simulink model "Model"  (R2023b)
settings: Solver=VariableStepAuto  StartTime=0.0  StopTime=20  RelTol=1e-3
InitFcn:
  | Parameters
values from neighbouring files (symbols this model uses):
  Area = 0.1    [Parameters.m]
  C_d = 1.05    [Parameters.m]
  cg_pos = [0.0 0 0.7]    [Parameters.m]
  ct_pos = [0 0 0.2]    [Parameters.m]
  Mass = 5    [Parameters.m]
undefined symbols (not defined in the file or in its folder): Continuous, R, Time
libraries: slpidlib x6, simulink_extras x5, sharedtransform x2, ctrlSharedLib x1, aerolibanim x1, shared6dof x1, vrlib x1, matrix_library x1
settings Model: Creator=zbyss  LastModifiedBy=zbyss

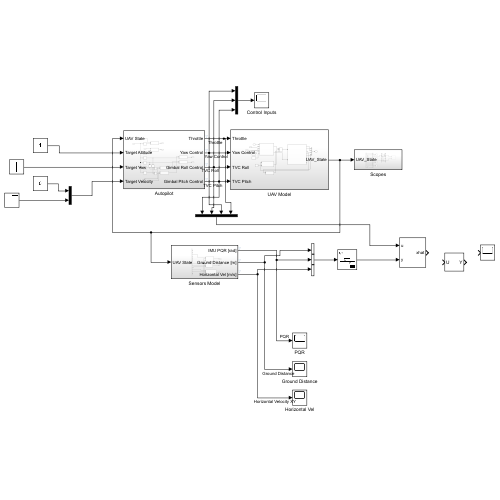
[thumbnail: Simulink's stored preview of the top-level diagram]
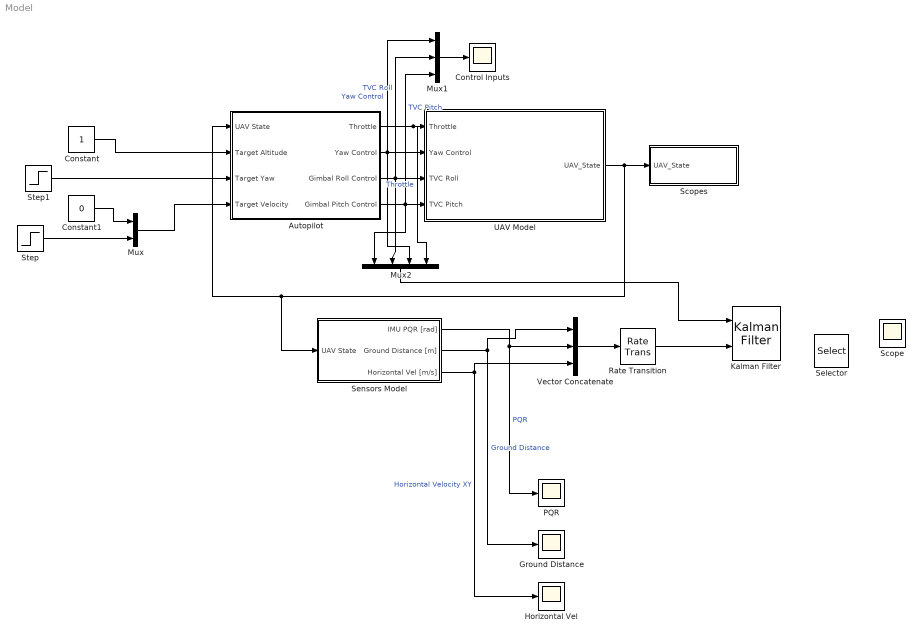
== system Model ==
  Autopilot : Subsystem
  Constant : Constant
  Constant1 : Constant  Value=0
  Control Inputs : Scope
  Ground Distance : Scope
  Horizontal Vel : Scope
  Kalman Filter : ctrlSharedLib/Kalman Filter  TimeDomain=Continuous-Time  UseCurrentEstimator=on  ModelSource=LTI State-Space Variable  ModelSourceVariable=UAV_ss  A=0.95  B=1  C=1  D=0  NumberOfStates=1  NumberOfInputs=1  NumberOfOutputs=1  InitialEstimateSource=Dialog  X0=0  P0=10  UseK=off  UseGH=off  NumberOfProcessNoiseInputs=1  G=1  TimeInvariantG=on  H=0  TimeInvariantH=on  Q=Q  TimeInvariantQ=on  R=R  TimeInvariantR=on  N=0  TimeInvariantN=on  AddInputPort=on  AddEnablePort=off  OutputEstimatedY=off  OutputP=off  Ts=-1
  Mux : Mux  Inputs=2
  Mux1 : Mux  Inputs=3
  Mux2 : Mux
  PQR : Scope
  Rate Transition : RateTransition
  Scope : Scope
  Scopes : Subsystem
  Selector : Selector  InputPortWidth=16  IndexOptions=Index vector (dialog)  Indices=[1 3]  OutputSizes=1
  Sensors Model : Subsystem
  Step : Step  Time=10  Before=-0.5  SampleTime=0
  Step1 : Step  Time=10  After=0  SampleTime=0
  UAV Model : Subsystem
  Vector Concatenate : Concatenate  NumInputs=3
  wires:
  Autopilot/1(Throttle) -> Mux2/4, UAV Model/1(Throttle)  "Throttle"
  Autopilot/2(Yaw Control) -> UAV Model/2(Yaw Control), Mux2/3, Mux1/1  "Yaw Control"
  Autopilot/3(Gimbal Roll Control) -> Mux2/2, Mux1/2, UAV Model/3(TVC Roll)  "TVC Roll"
  Autopilot/4(Gimbal Pitch Control) -> Mux2/1, Mux1/3, UAV Model/4(TVC Pitch)  "TVC Pitch"
  UAV Model/1(UAV_State) -> Sensors Model/1(UAV State), Autopilot/1(UAV State), Scopes/1(UAV_State)
  Constant/1 -> Autopilot/2(Target Altitude)
  Constant1/1 -> Mux/1
  Step/1 -> Mux/2
  Mux/1 -> Autopilot/4(Target Velocity)
  Sensors Model/1(IMU PQR [rad]) -> Vector Concatenate/2, PQR/1  "PQR"
  Sensors Model/2(Ground Distance [m]) -> Vector Concatenate/1, Ground Distance/1  "Ground Distance"
  Sensors Model/3(Horizontal Vel [m/s]) -> Vector Concatenate/3, Horizontal Vel/1  "Horizontal Velocity XY"
  Mux1/1 -> Control Inputs/1
  Step1/1 -> Autopilot/3(Target Yaw)
  Vector Concatenate/1 -> Rate Transition/1
  Mux2/1 -> Kalman Filter/1
  Rate Transition/1 -> Kalman Filter/2

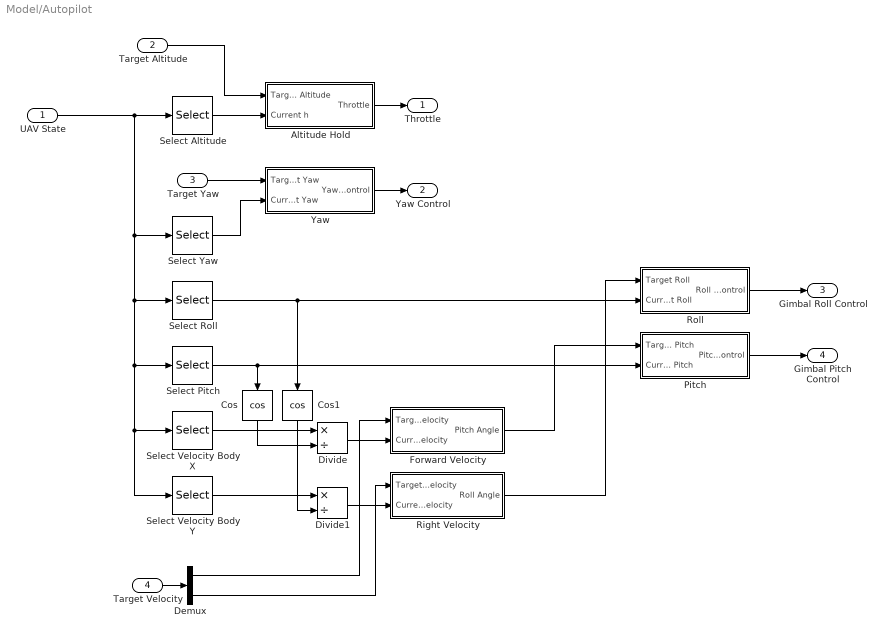
== system Model/Autopilot ==
  UAV State : Inport
  Target Altitude : Inport  Port=2
  Target Yaw : Inport  Port=3
  Target Velocity : Inport  Port=4
  Altitude Hold : Subsystem
  Cos : Trigonometry  Operator=cos
  Cos1 : Trigonometry  Operator=cos
  Demux : Demux  Outputs=2
  Divide : Product  Inputs=*/
  Divide1 : Product  Inputs=*/
  Forward Velocity : Subsystem
  Pitch : Subsystem
  Right Velocity : Subsystem
  Roll : Subsystem
  Select Altitude : Selector  InputPortWidth=12  IndexOptions=Index vector (dialog)  Indices=[3]  OutputSizes=1
  Select Pitch : Selector  InputPortWidth=12  IndexOptions=Index vector (dialog)  Indices=[8]  OutputSizes=1
  Select Roll : Selector  InputPortWidth=12  IndexOptions=Index vector (dialog)  Indices=[7]  OutputSizes=1
  Select Velocity Body X : Selector  InputPortWidth=12  IndexOptions=Index vector (dialog)  Indices=[10]  OutputSizes=1
  Select Velocity Body Y : Selector  InputPortWidth=12  IndexOptions=Index vector (dialog)  Indices=[11]  OutputSizes=1
  Select Yaw : Selector  InputPortWidth=12  IndexOptions=Index vector (dialog)  Indices=[9]  OutputSizes=1
  Yaw : Subsystem
  Throttle : Outport
  Yaw Control : Outport  Port=2
  Gimbal Roll Control : Outport  Port=3
  Gimbal Pitch Control : Outport  Port=4
  wires:
  Target Altitude/1 -> Altitude Hold/1(Target Altitude)
  Select Altitude/1 -> Altitude Hold/2(Current h)
  UAV State/1 -> Select Roll/1, Select Velocity Body Y/1, Select Velocity Body X/1, Select Pitch/1, Select Yaw/1, Select Altitude/1
  Altitude Hold/1(Throttle) -> Throttle/1
  Target Yaw/1 -> Yaw/1(Target Yaw)
  Select Yaw/1 -> Yaw/2(Current Yaw)
  Yaw/1(Yaw Control) -> Yaw Control/1
  Pitch/1(Pitch Control) -> Gimbal Pitch Control/1
  Select Pitch/1 -> Cos/1, Pitch/2(Current Pitch)
  Roll/1(Roll Control) -> Gimbal Roll Control/1
  Select Roll/1 -> Cos1/1, Roll/2(Current Roll)
  Target Velocity/1 -> Demux/1
  Select Velocity Body X/1 -> Divide/1
  Cos/1 -> Divide/2
  Divide/1 -> Forward Velocity/2(Current Velocity)
  Demux/1 -> Forward Velocity/1(Target Velocity)
  Forward Velocity/1(Pitch Angle) -> Pitch/1(Target Pitch)
  Right Velocity/1(Roll Angle) -> Roll/1(Target Roll)
  Demux/2 -> Right Velocity/1(Target Velocity)
  Divide1/1 -> Right Velocity/2(Current Velocity)
  Select Velocity Body Y/1 -> Divide1/1
  Cos1/1 -> Divide1/2

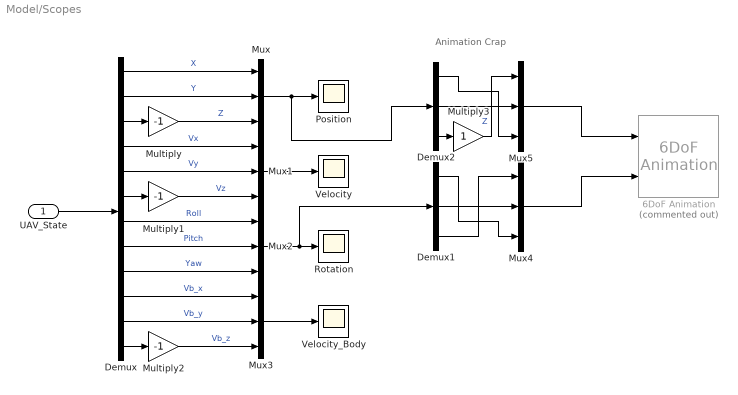
== system Model/Scopes ==
  note: Animation Crap
  UAV_State : Inport
  6DoF Animation : aerolibanim/6DoF Animation  Commented=on  u1=[-50 50 -50 50 -50 50]  u2=0.1  u3=1.0  u4=[10 0 0]  u5=Fly alongside  u6=[1 0 10]  u7=10  u8=on
  Demux : Demux  Outputs=12
  Demux1 : Demux  Outputs=3
  Demux2 : Demux  Outputs=3
  Multiply : Gain  Gain=-1
  Multiply1 : Gain  Gain=-1
  Multiply2 : Gain  Gain=-1
  Multiply3 : Gain
  Mux{,1..5} (6 alike) : Mux  Inputs=3
  Position : Scope
  Rotation : Scope
  Velocity : Scope
  Velocity_Body : Scope
  wires:
  UAV_State/1 -> Demux/1
  Demux/1 -> Mux/1  "X"
  Demux/2 -> Mux/2  "Y"
  Demux/3 -> Multiply/1
  Mux/1 -> Demux2/1, Position/1
  Demux/4 -> Mux1/1  "Vx"
  Demux/5 -> Mux1/2  "Vy"
  Demux/6 -> Multiply1/1
  Mux1/1 -> Velocity/1
  Demux/7 -> Mux2/1  "Roll"
  Demux/8 -> Mux2/2  "Pitch"
  Demux/9 -> Mux2/3  "Yaw"
  Multiply/1 -> Mux/3  "Z"
  Multiply1/1 -> Mux1/3  "Vz"
  Mux3/1 -> Velocity_Body/1
  Demux/12 -> Multiply2/1
  Multiply2/1 -> Mux3/3  "Vb_z"
  Demux/11 -> Mux3/2  "Vb_y"
  Demux/10 -> Mux3/1  "Vb_x"
  Mux2/1 -> Demux1/1, Rotation/1
  Mux4/1 -> 6DoF Animation/2
  Demux1/3 -> Mux4/1
  Demux1/2 -> Mux4/2
  Demux1/1 -> Mux4/3
  Demux2/2 -> Mux5/2
  Demux2/1 -> Mux5/3
  Demux2/3 -> Multiply3/1
  Multiply3/1 -> Mux5/1  "Z"
  Mux5/1 -> 6DoF Animation/1

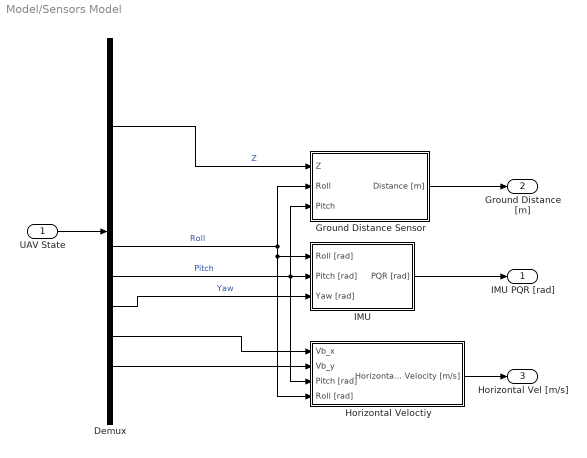
== system Model/Sensors Model ==
  UAV State : Inport
  Demux : Demux  Outputs=12
  Ground Distance Sensor : Subsystem
  Horizontal Veloctiy : Subsystem
  IMU : Subsystem
  IMU PQR [rad] : Outport
  Ground Distance [m] : Outport  Port=2
  Horizontal Vel [m/s] : Outport  Port=3
  wires:
  UAV State/1 -> Demux/1
  Demux/7 -> Horizontal Veloctiy/4(Roll [rad]), IMU/1(Roll [rad]), Ground Distance Sensor/2(Roll)  "Roll"
  Demux/8 -> Horizontal Veloctiy/3(Pitch [rad]), Ground Distance Sensor/3(Pitch), IMU/2(Pitch [rad])  "Pitch"
  Demux/9 -> IMU/3(Yaw [rad])  "Yaw"
  IMU/1(PQR [rad]) -> IMU PQR [rad]/1
  Demux/3 -> Ground Distance Sensor/1(Z)  "Z"
  Ground Distance Sensor/1(Distance [m]) -> Ground Distance [m]/1
  Demux/10 -> Horizontal Veloctiy/1(Vb_x)
  Demux/11 -> Horizontal Veloctiy/2(Vb_y)
  Horizontal Veloctiy/1(Horizontal Velocity [m/s]) -> Horizontal Vel [m/s]/1

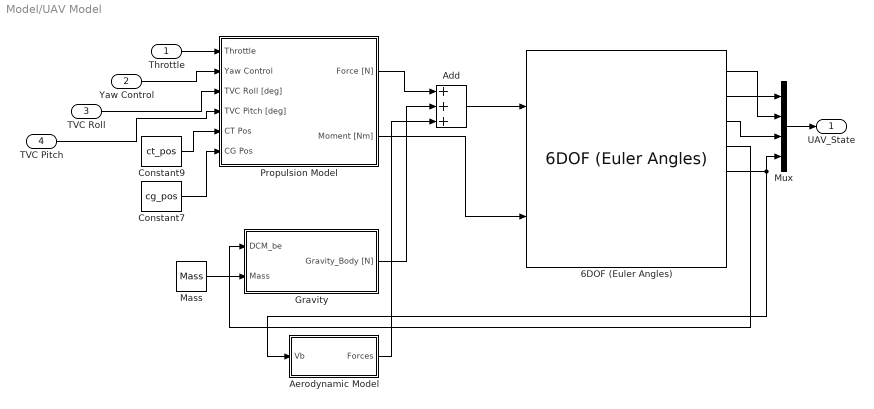
== system Model/UAV Model ==
  Throttle : Inport
  Yaw Control : Inport  Port=2
  TVC Roll : Inport  Port=3
  TVC Pitch : Inport  Port=4
  6DOF (Euler Angles) : shared6dof/6DOF (Euler Angles)  units=Metric (MKS)  mtype=Fixed  rep=Euler Angles  xme_0=[0 0 0]  Vm_0=[0 0 0]  eul_0=[0 0 0]  pm_0=[0 0 0]  mass_0=Mass  mass_e=0.5  mass_f=2.0  inertia=eye(3)  inertia_e=eye(3)  inertia_f=2*eye(3)  k_quat=1.0  vre_flag=on  abi_flag=off  aMode=0  xme_statename=''  Vm_statename=''  eul_statename=''  quat_statename=''  pm_statename=''  mass_statename=''
  Add : Sum  Inputs=+++
  Aerodynamic Model : Subsystem
  Constant7 : Constant  Value=cg_pos
  Constant9 : Constant  Value=ct_pos
  Gravity : Subsystem
  Mass : Constant  Value=Mass
  Mux : Mux
  Propulsion Model : Subsystem
  UAV_State : Outport
  wires:
  Propulsion Model/1(Force [N]) -> Add/1
  Add/1 -> 6DOF (Euler Angles)/1
  TVC Roll/1 -> Propulsion Model/3(TVC Roll [deg])
  Throttle/1 -> Propulsion Model/1(Throttle)
  Gravity/1(Gravity_Body [N]) -> Add/2
  Propulsion Model/2(Moment [Nm]) -> 6DOF (Euler Angles)/2
  Constant9/1 -> Propulsion Model/5(CT Pos)
  Constant7/1 -> Propulsion Model/6(CG Pos)
  Mass/1 -> Gravity/2(Mass)
  6DOF (Euler Angles)/4 -> Gravity/1(DCM_be)
  Yaw Control/1 -> Propulsion Model/2(Yaw Control)
  6DOF (Euler Angles)/3 -> Mux/3
  6DOF (Euler Angles)/2 -> Mux/1
  Mux/1 -> UAV_State/1
  TVC Pitch/1 -> Propulsion Model/4(TVC Pitch [deg])
  6DOF (Euler Angles)/1 -> Mux/2
  6DOF (Euler Angles)/5 -> Aerodynamic Model/1(Vb), Mux/4
  Aerodynamic Model/1(Forces) -> Add/3

== system Model/Autopilot/Altitude Hold ==
  Target Altitude : Inport
  Current h : Inport  Port=2
  Altitude Hold PID : slpidlib/PID Controller  Controller=PID  Form=Parallel  TimeDomain=Continuous-time  UseExternalTs=off  SampleTime=-1  IntegratorMethod=Forward Euler  FilterMethod=Forward Euler  ControllerParametersSource=internal  P=1.20920987907462  I=0.107771167125322  UseKiTs=off  D=3.01454491123333  N=1745.9050909753  UseFilter=on  TunerSelectOption=Transfer Function Based (PID Tuner App)  InitialConditionSource=internal  InitialConditionForIntegrator=0  InitialConditionForFilter=0  DifferentiatorICPrevScaledInput=0  ExternalReset=none  TrackingMode=off  Kt=1  LimitOutput=off  SatLimitsSource=internal  UpperSaturationLimit=inf  LowerSaturationLimit=-inf  LinearizeAsGain=on  AntiWindupMode=none  Kb=1  LimitIntegrator=off  UpperIntegratorSaturationLimit=inf  LowerIntegratorSaturationLimit=-inf  POutMin=[]  POutMax=[]  IOutMin=[]  IOutMax=[]  DOutMin=[]  DOutMax=[]  NOutMin=[]  NOutMax=[]  SumOutMin=[]  SumOutMax=[]  SaturationOutMin=[]  SaturationOutMax=[]  PParamMin=[]  PParamMax=[]  IParamMin=[]  IParamMax=[]  DParamMin=[]  DParamMax=[]  NParamMin=[]  NParamMax=[]  KbParamMin=[]  KbParamMax=[]  KtParamMin=[]  KtParamMax=[]  KbOutMin=[]  KbOutMax=[]  KtOutMin=[]  KtOutMax=[]  IntegratorOutMin=[]  IntegratorOutMax=[]  FilterOutMin=[]  FilterOutMax=[]  SumI1OutMin=[]  SumI1OutMax=[]  SumI2OutMin=[]  SumI2OutMax=[]  SumI3OutMin=[]  SumI3OutMax=[]  SumI4OutMin=[]  SumI4OutMax=[]  SumDOutMin=[]  SumDOutMax=[]  DifferentiatorOutMin=[]  DifferentiatorOutMax=[]  FilterDiffOutCoefMin=[]  FilterDiffOutCoefMax=[]  ReciprocalOutMin=[]  ReciprocalOutMax=[]  SumDenOutMin=[]  SumDenOutMax=[]  SumNumOutMin=[]  SumNumOutMax=[]  DivideOutMin=[]  DivideOutMax=[]  UdiffTsProdOutMin=[]  UdiffTsProdOutMax=[]  NTsProdOutMin=[]  NTsProdOutMax=[]  UintegralTsProdOutMin=[]  UintegralTsProdOutMax=[]  UngainTsProdOutMin=[]  UngainTsProdOutMax=[]  ClampingZeroOutDataTypeStr=Inherit: Inherit via back propagation  ClampingZeroOutMin=[]  ClampingZeroOutMax=[]  FilterDenConstantOutDataTypeStr=Inherit: Inherit via back propagation  FilterDenConstantOutMin=[]  FilterDenConstantOutMax=[]  PCopyOutDataTypeStr=Inherit: Inherit via back propagation  PCopyOutMin=[]  PCopyOutMax=[]  NCopyOutDataTypeStr=Inherit: Inherit via back propagation  NCopyOutMin=[]  NCopyOutMax=[]  IntegratorContinuousStateAttributes=''  IntegratorStateMustResolveToSignalObject=off  IntegratorRTWStateStorageClass=Auto  FilterContinuousStateAttributes=''  FilterStateMustResolveToSignalObject=off  FilterRTWStateStorageClass=Auto  ParallelPVariant=InternalParameters  IdealPVariant=Disabled  IVariant=InternalParameters  DVariant=InternalParameters  IntegratorVariant=Continuous  SatVariant=Disabled  AWVariant=Passthrough  PCopyVariant=Disabled  TRVariant=Disabled  FdbkBlocksVariant=Forward  IdealPFdbkVariant=Disabled  SatFdbkVariant=Disabled  DerivativeFilterVariant=ContFilter  NVariant=InternalParameters  NCopyVariant=Disabled  FilterICVariant=InternalICsFilter  IntegratorICVariant=InternalICs  ExternalResetVariant=Disabled  TRSumVariant=Passthrough  SumFdbkVariant=Disabled  SumVariant=Sum_PID  TsampFilterVariant=InternalTs  TsampNgainVariant=Passthrough  TsampIntegralVariant=Disabled_SignalSpec  ExternalSaturationOutDataTypeStr=Inherit: Same as second input
  Multiply : Gain  Gain=-1
  Saturation : Saturate  UpperLimit=1  LowerLimit=0
  Sum : Sum  Inputs=|+-
  Throttle : Outport
  wires:
  Sum/1 -> Altitude Hold PID/1
  Target Altitude/1 -> Sum/1
  Current h/1 -> Multiply/1
  Altitude Hold PID/1 -> Saturation/1
  Multiply/1 -> Sum/2
  Saturation/1 -> Throttle/1

== system Model/Autopilot/Forward Velocity ==
  Target Velocity : Inport
  Current Velocity : Inport  Port=2
  Gain : Gain  Gain=-1
  PID Controller : slpidlib/PID Controller  Controller=PID  Form=Parallel  TimeDomain=Continuous-time  UseExternalTs=off  SampleTime=-1  IntegratorMethod=Forward Euler  FilterMethod=Forward Euler  ControllerParametersSource=internal  P=5  I=1  UseKiTs=off  D=0  N=100  UseFilter=on  TunerSelectOption=Transfer Function Based (PID Tuner App)  InitialConditionSource=internal  InitialConditionForIntegrator=0  InitialConditionForFilter=0  DifferentiatorICPrevScaledInput=0  ExternalReset=none  TrackingMode=off  Kt=1  LimitOutput=off  SatLimitsSource=internal  UpperSaturationLimit=inf  LowerSaturationLimit=-inf  LinearizeAsGain=on  AntiWindupMode=none  Kb=1  LimitIntegrator=off  UpperIntegratorSaturationLimit=inf  LowerIntegratorSaturationLimit=-inf  POutMin=[]  POutMax=[]  IOutMin=[]  IOutMax=[]  DOutMin=[]  DOutMax=[]  NOutMin=[]  NOutMax=[]  SumOutMin=[]  SumOutMax=[]  SaturationOutMin=[]  SaturationOutMax=[]  PParamMin=[]  PParamMax=[]  IParamMin=[]  IParamMax=[]  DParamMin=[]  DParamMax=[]  NParamMin=[]  NParamMax=[]  KbParamMin=[]  KbParamMax=[]  KtParamMin=[]  KtParamMax=[]  KbOutMin=[]  KbOutMax=[]  KtOutMin=[]  KtOutMax=[]  IntegratorOutMin=[]  IntegratorOutMax=[]  FilterOutMin=[]  FilterOutMax=[]  SumI1OutMin=[]  SumI1OutMax=[]  SumI2OutMin=[]  SumI2OutMax=[]  SumI3OutMin=[]  SumI3OutMax=[]  SumI4OutMin=[]  SumI4OutMax=[]  SumDOutMin=[]  SumDOutMax=[]  DifferentiatorOutMin=[]  DifferentiatorOutMax=[]  FilterDiffOutCoefMin=[]  FilterDiffOutCoefMax=[]  ReciprocalOutMin=[]  ReciprocalOutMax=[]  SumDenOutMin=[]  SumDenOutMax=[]  SumNumOutMin=[]  SumNumOutMax=[]  DivideOutMin=[]  DivideOutMax=[]  UdiffTsProdOutMin=[]  UdiffTsProdOutMax=[]  NTsProdOutMin=[]  NTsProdOutMax=[]  UintegralTsProdOutMin=[]  UintegralTsProdOutMax=[]  UngainTsProdOutMin=[]  UngainTsProdOutMax=[]  ClampingZeroOutDataTypeStr=Inherit: Inherit via back propagation  ClampingZeroOutMin=[]  ClampingZeroOutMax=[]  FilterDenConstantOutDataTypeStr=Inherit: Inherit via back propagation  FilterDenConstantOutMin=[]  FilterDenConstantOutMax=[]  PCopyOutDataTypeStr=Inherit: Inherit via back propagation  PCopyOutMin=[]  PCopyOutMax=[]  NCopyOutDataTypeStr=Inherit: Inherit via back propagation  NCopyOutMin=[]  NCopyOutMax=[]  IntegratorContinuousStateAttributes=''  IntegratorStateMustResolveToSignalObject=off  IntegratorRTWStateStorageClass=Auto  FilterContinuousStateAttributes=''  FilterStateMustResolveToSignalObject=off  FilterRTWStateStorageClass=Auto  ParallelPVariant=InternalParameters  IdealPVariant=Disabled  IVariant=InternalParameters  DVariant=InternalParameters  IntegratorVariant=Continuous  SatVariant=Disabled  AWVariant=Passthrough  PCopyVariant=Disabled  TRVariant=Disabled  FdbkBlocksVariant=Forward  IdealPFdbkVariant=Disabled  SatFdbkVariant=Disabled  DerivativeFilterVariant=ContFilter  NVariant=InternalParameters  NCopyVariant=Disabled  FilterICVariant=InternalICsFilter  IntegratorICVariant=InternalICs  ExternalResetVariant=Disabled  TRSumVariant=Passthrough  SumFdbkVariant=Disabled  SumVariant=Sum_PID  TsampFilterVariant=InternalTs  TsampNgainVariant=Passthrough  TsampIntegralVariant=Disabled_SignalSpec  ExternalSaturationOutDataTypeStr=Inherit: Same as second input
  Saturation : Saturate  UpperLimit=5  LowerLimit=-5
  Sum : Sum  Inputs=|+-
  Pitch Angle : Outport
  wires:
  Target Velocity/1 -> Sum/1
  Current Velocity/1 -> Sum/2
  Sum/1 -> PID Controller/1
  PID Controller/1 -> Gain/1
  Saturation/1 -> Pitch Angle/1
  Gain/1 -> Saturation/1

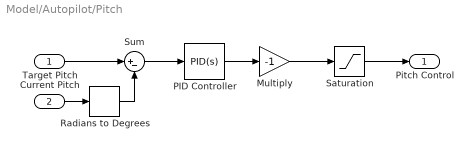
== system Model/Autopilot/Pitch ==
  Target Pitch : Inport
  Current Pitch : Inport  Port=2
  Multiply : Gain  Gain=-1
  PID Controller : slpidlib/PID Controller  Controller=PID  Form=Parallel  TimeDomain=Continuous-time  UseExternalTs=off  SampleTime=-1  IntegratorMethod=Forward Euler  FilterMethod=Forward Euler  ControllerParametersSource=internal  P=2  I=1  UseKiTs=off  D=1  N=100  UseFilter=on  TunerSelectOption=Transfer Function Based (PID Tuner App)  InitialConditionSource=internal  InitialConditionForIntegrator=0  InitialConditionForFilter=0  DifferentiatorICPrevScaledInput=0  ExternalReset=none  TrackingMode=off  Kt=1  LimitOutput=off  SatLimitsSource=internal  UpperSaturationLimit=inf  LowerSaturationLimit=-inf  LinearizeAsGain=on  AntiWindupMode=none  Kb=1  LimitIntegrator=off  UpperIntegratorSaturationLimit=inf  LowerIntegratorSaturationLimit=-inf  POutMin=[]  POutMax=[]  IOutMin=[]  IOutMax=[]  DOutMin=[]  DOutMax=[]  NOutMin=[]  NOutMax=[]  SumOutMin=[]  SumOutMax=[]  SaturationOutMin=[]  SaturationOutMax=[]  PParamMin=[]  PParamMax=[]  IParamMin=[]  IParamMax=[]  DParamMin=[]  DParamMax=[]  NParamMin=[]  NParamMax=[]  KbParamMin=[]  KbParamMax=[]  KtParamMin=[]  KtParamMax=[]  KbOutMin=[]  KbOutMax=[]  KtOutMin=[]  KtOutMax=[]  IntegratorOutMin=[]  IntegratorOutMax=[]  FilterOutMin=[]  FilterOutMax=[]  SumI1OutMin=[]  SumI1OutMax=[]  SumI2OutMin=[]  SumI2OutMax=[]  SumI3OutMin=[]  SumI3OutMax=[]  SumI4OutMin=[]  SumI4OutMax=[]  SumDOutMin=[]  SumDOutMax=[]  DifferentiatorOutMin=[]  DifferentiatorOutMax=[]  FilterDiffOutCoefMin=[]  FilterDiffOutCoefMax=[]  ReciprocalOutMin=[]  ReciprocalOutMax=[]  SumDenOutMin=[]  SumDenOutMax=[]  SumNumOutMin=[]  SumNumOutMax=[]  DivideOutMin=[]  DivideOutMax=[]  UdiffTsProdOutMin=[]  UdiffTsProdOutMax=[]  NTsProdOutMin=[]  NTsProdOutMax=[]  UintegralTsProdOutMin=[]  UintegralTsProdOutMax=[]  UngainTsProdOutMin=[]  UngainTsProdOutMax=[]  ClampingZeroOutDataTypeStr=Inherit: Inherit via back propagation  ClampingZeroOutMin=[]  ClampingZeroOutMax=[]  FilterDenConstantOutDataTypeStr=Inherit: Inherit via back propagation  FilterDenConstantOutMin=[]  FilterDenConstantOutMax=[]  PCopyOutDataTypeStr=Inherit: Inherit via back propagation  PCopyOutMin=[]  PCopyOutMax=[]  NCopyOutDataTypeStr=Inherit: Inherit via back propagation  NCopyOutMin=[]  NCopyOutMax=[]  IntegratorContinuousStateAttributes=''  IntegratorStateMustResolveToSignalObject=off  IntegratorRTWStateStorageClass=Auto  FilterContinuousStateAttributes=''  FilterStateMustResolveToSignalObject=off  FilterRTWStateStorageClass=Auto  ParallelPVariant=InternalParameters  IdealPVariant=Disabled  IVariant=InternalParameters  DVariant=InternalParameters  IntegratorVariant=Continuous  SatVariant=Disabled  AWVariant=Passthrough  PCopyVariant=Disabled  TRVariant=Disabled  FdbkBlocksVariant=Forward  IdealPFdbkVariant=Disabled  SatFdbkVariant=Disabled  DerivativeFilterVariant=ContFilter  NVariant=InternalParameters  NCopyVariant=Disabled  FilterICVariant=InternalICsFilter  IntegratorICVariant=InternalICs  ExternalResetVariant=Disabled  TRSumVariant=Passthrough  SumFdbkVariant=Disabled  SumVariant=Sum_PID  TsampFilterVariant=InternalTs  TsampNgainVariant=Passthrough  TsampIntegralVariant=Disabled_SignalSpec  ExternalSaturationOutDataTypeStr=Inherit: Same as second input
  Radians to Degrees : simulink_extras/Transformations/Radians to Degrees
  Saturation : Saturate  UpperLimit=15  LowerLimit=-15
  Sum : Sum  Inputs=|+-
  Pitch Control : Outport
  wires:
  Target Pitch/1 -> Sum/1
  PID Controller/1 -> Multiply/1
  Current Pitch/1 -> Radians to Degrees/1
  Sum/1 -> PID Controller/1
  Saturation/1 -> Pitch Control/1
  Multiply/1 -> Saturation/1
  Radians to Degrees/1 -> Sum/2

== system Model/Autopilot/Right Velocity ==
  Target Velocity : Inport
  Current Velocity : Inport  Port=2
  PID Controller : slpidlib/PID Controller  Controller=PID  Form=Parallel  TimeDomain=Continuous-time  UseExternalTs=off  SampleTime=-1  IntegratorMethod=Forward Euler  FilterMethod=Forward Euler  ControllerParametersSource=internal  P=5  I=1  UseKiTs=off  D=0  N=100  UseFilter=on  TunerSelectOption=Transfer Function Based (PID Tuner App)  InitialConditionSource=internal  InitialConditionForIntegrator=0  InitialConditionForFilter=0  DifferentiatorICPrevScaledInput=0  ExternalReset=none  TrackingMode=off  Kt=1  LimitOutput=off  SatLimitsSource=internal  UpperSaturationLimit=inf  LowerSaturationLimit=-inf  LinearizeAsGain=on  AntiWindupMode=none  Kb=1  LimitIntegrator=off  UpperIntegratorSaturationLimit=inf  LowerIntegratorSaturationLimit=-inf  POutMin=[]  POutMax=[]  IOutMin=[]  IOutMax=[]  DOutMin=[]  DOutMax=[]  NOutMin=[]  NOutMax=[]  SumOutMin=[]  SumOutMax=[]  SaturationOutMin=[]  SaturationOutMax=[]  PParamMin=[]  PParamMax=[]  IParamMin=[]  IParamMax=[]  DParamMin=[]  DParamMax=[]  NParamMin=[]  NParamMax=[]  KbParamMin=[]  KbParamMax=[]  KtParamMin=[]  KtParamMax=[]  KbOutMin=[]  KbOutMax=[]  KtOutMin=[]  KtOutMax=[]  IntegratorOutMin=[]  IntegratorOutMax=[]  FilterOutMin=[]  FilterOutMax=[]  SumI1OutMin=[]  SumI1OutMax=[]  SumI2OutMin=[]  SumI2OutMax=[]  SumI3OutMin=[]  SumI3OutMax=[]  SumI4OutMin=[]  SumI4OutMax=[]  SumDOutMin=[]  SumDOutMax=[]  DifferentiatorOutMin=[]  DifferentiatorOutMax=[]  FilterDiffOutCoefMin=[]  FilterDiffOutCoefMax=[]  ReciprocalOutMin=[]  ReciprocalOutMax=[]  SumDenOutMin=[]  SumDenOutMax=[]  SumNumOutMin=[]  SumNumOutMax=[]  DivideOutMin=[]  DivideOutMax=[]  UdiffTsProdOutMin=[]  UdiffTsProdOutMax=[]  NTsProdOutMin=[]  NTsProdOutMax=[]  UintegralTsProdOutMin=[]  UintegralTsProdOutMax=[]  UngainTsProdOutMin=[]  UngainTsProdOutMax=[]  ClampingZeroOutDataTypeStr=Inherit: Inherit via back propagation  ClampingZeroOutMin=[]  ClampingZeroOutMax=[]  FilterDenConstantOutDataTypeStr=Inherit: Inherit via back propagation  FilterDenConstantOutMin=[]  FilterDenConstantOutMax=[]  PCopyOutDataTypeStr=Inherit: Inherit via back propagation  PCopyOutMin=[]  PCopyOutMax=[]  NCopyOutDataTypeStr=Inherit: Inherit via back propagation  NCopyOutMin=[]  NCopyOutMax=[]  IntegratorContinuousStateAttributes=''  IntegratorStateMustResolveToSignalObject=off  IntegratorRTWStateStorageClass=Auto  FilterContinuousStateAttributes=''  FilterStateMustResolveToSignalObject=off  FilterRTWStateStorageClass=Auto  ParallelPVariant=InternalParameters  IdealPVariant=Disabled  IVariant=InternalParameters  DVariant=InternalParameters  IntegratorVariant=Continuous  SatVariant=Disabled  AWVariant=Passthrough  PCopyVariant=Disabled  TRVariant=Disabled  FdbkBlocksVariant=Forward  IdealPFdbkVariant=Disabled  SatFdbkVariant=Disabled  DerivativeFilterVariant=ContFilter  NVariant=InternalParameters  NCopyVariant=Disabled  FilterICVariant=InternalICsFilter  IntegratorICVariant=InternalICs  ExternalResetVariant=Disabled  TRSumVariant=Passthrough  SumFdbkVariant=Disabled  SumVariant=Sum_PID  TsampFilterVariant=InternalTs  TsampNgainVariant=Passthrough  TsampIntegralVariant=Disabled_SignalSpec  ExternalSaturationOutDataTypeStr=Inherit: Same as second input
  Saturation : Saturate  UpperLimit=5  LowerLimit=-5
  Sum : Sum  Inputs=|+-
  Roll Angle : Outport
  wires:
  Target Velocity/1 -> Sum/1
  Current Velocity/1 -> Sum/2
  Sum/1 -> PID Controller/1
  PID Controller/1 -> Saturation/1
  Saturation/1 -> Roll Angle/1

== system Model/Autopilot/Roll ==
  Target Roll : Inport
  Current Roll : Inport  Port=2
  Multiply : Gain  Gain=-1
  PID Controller : slpidlib/PID Controller  Controller=PID  Form=Parallel  TimeDomain=Continuous-time  UseExternalTs=off  SampleTime=-1  IntegratorMethod=Forward Euler  FilterMethod=Forward Euler  ControllerParametersSource=internal  P=1  I=1  UseKiTs=off  D=1  N=100  UseFilter=on  TunerSelectOption=Transfer Function Based (PID Tuner App)  InitialConditionSource=internal  InitialConditionForIntegrator=0  InitialConditionForFilter=0  DifferentiatorICPrevScaledInput=0  ExternalReset=none  TrackingMode=off  Kt=1  LimitOutput=off  SatLimitsSource=internal  UpperSaturationLimit=inf  LowerSaturationLimit=-inf  LinearizeAsGain=on  AntiWindupMode=none  Kb=1  LimitIntegrator=off  UpperIntegratorSaturationLimit=inf  LowerIntegratorSaturationLimit=-inf  POutMin=[]  POutMax=[]  IOutMin=[]  IOutMax=[]  DOutMin=[]  DOutMax=[]  NOutMin=[]  NOutMax=[]  SumOutMin=[]  SumOutMax=[]  SaturationOutMin=[]  SaturationOutMax=[]  PParamMin=[]  PParamMax=[]  IParamMin=[]  IParamMax=[]  DParamMin=[]  DParamMax=[]  NParamMin=[]  NParamMax=[]  KbParamMin=[]  KbParamMax=[]  KtParamMin=[]  KtParamMax=[]  KbOutMin=[]  KbOutMax=[]  KtOutMin=[]  KtOutMax=[]  IntegratorOutMin=[]  IntegratorOutMax=[]  FilterOutMin=[]  FilterOutMax=[]  SumI1OutMin=[]  SumI1OutMax=[]  SumI2OutMin=[]  SumI2OutMax=[]  SumI3OutMin=[]  SumI3OutMax=[]  SumI4OutMin=[]  SumI4OutMax=[]  SumDOutMin=[]  SumDOutMax=[]  DifferentiatorOutMin=[]  DifferentiatorOutMax=[]  FilterDiffOutCoefMin=[]  FilterDiffOutCoefMax=[]  ReciprocalOutMin=[]  ReciprocalOutMax=[]  SumDenOutMin=[]  SumDenOutMax=[]  SumNumOutMin=[]  SumNumOutMax=[]  DivideOutMin=[]  DivideOutMax=[]  UdiffTsProdOutMin=[]  UdiffTsProdOutMax=[]  NTsProdOutMin=[]  NTsProdOutMax=[]  UintegralTsProdOutMin=[]  UintegralTsProdOutMax=[]  UngainTsProdOutMin=[]  UngainTsProdOutMax=[]  ClampingZeroOutDataTypeStr=Inherit: Inherit via back propagation  ClampingZeroOutMin=[]  ClampingZeroOutMax=[]  FilterDenConstantOutDataTypeStr=Inherit: Inherit via back propagation  FilterDenConstantOutMin=[]  FilterDenConstantOutMax=[]  PCopyOutDataTypeStr=Inherit: Inherit via back propagation  PCopyOutMin=[]  PCopyOutMax=[]  NCopyOutDataTypeStr=Inherit: Inherit via back propagation  NCopyOutMin=[]  NCopyOutMax=[]  IntegratorContinuousStateAttributes=''  IntegratorStateMustResolveToSignalObject=off  IntegratorRTWStateStorageClass=Auto  FilterContinuousStateAttributes=''  FilterStateMustResolveToSignalObject=off  FilterRTWStateStorageClass=Auto  ParallelPVariant=InternalParameters  IdealPVariant=Disabled  IVariant=InternalParameters  DVariant=InternalParameters  IntegratorVariant=Continuous  SatVariant=Disabled  AWVariant=Passthrough  PCopyVariant=Disabled  TRVariant=Disabled  FdbkBlocksVariant=Forward  IdealPFdbkVariant=Disabled  SatFdbkVariant=Disabled  DerivativeFilterVariant=ContFilter  NVariant=InternalParameters  NCopyVariant=Disabled  FilterICVariant=InternalICsFilter  IntegratorICVariant=InternalICs  ExternalResetVariant=Disabled  TRSumVariant=Passthrough  SumFdbkVariant=Disabled  SumVariant=Sum_PID  TsampFilterVariant=InternalTs  TsampNgainVariant=Passthrough  TsampIntegralVariant=Disabled_SignalSpec  ExternalSaturationOutDataTypeStr=Inherit: Same as second input
  Radians to Degrees : simulink_extras/Transformations/Radians to Degrees
  Saturation : Saturate  UpperLimit=15  LowerLimit=-15
  Sum : Sum  Inputs=|+-
  Roll Control : Outport
  wires:
  Target Roll/1 -> Sum/1
  PID Controller/1 -> Multiply/1
  Current Roll/1 -> Radians to Degrees/1
  Radians to Degrees/1 -> Sum/2
  Sum/1 -> PID Controller/1
  Saturation/1 -> Roll Control/1
  Multiply/1 -> Saturation/1

== system Model/Autopilot/Yaw ==
  Target Yaw : Inport
  Current Yaw : Inport  Port=2
  PID Controller : slpidlib/PID Controller  Controller=PID  Form=Parallel  TimeDomain=Continuous-time  UseExternalTs=off  SampleTime=-1  IntegratorMethod=Forward Euler  FilterMethod=Forward Euler  ControllerParametersSource=internal  P=0.042797411577694  I=0.000605883707407974  UseKiTs=off  D=0.5015154023923  N=234.053751783226  UseFilter=on  TunerSelectOption=Transfer Function Based (PID Tuner App)  InitialConditionSource=internal  InitialConditionForIntegrator=0  InitialConditionForFilter=0  DifferentiatorICPrevScaledInput=0  ExternalReset=none  TrackingMode=off  Kt=1  LimitOutput=off  SatLimitsSource=internal  UpperSaturationLimit=inf  LowerSaturationLimit=-inf  LinearizeAsGain=on  AntiWindupMode=none  Kb=1  LimitIntegrator=off  UpperIntegratorSaturationLimit=inf  LowerIntegratorSaturationLimit=-inf  POutMin=[]  POutMax=[]  IOutMin=[]  IOutMax=[]  DOutMin=[]  DOutMax=[]  NOutMin=[]  NOutMax=[]  SumOutMin=[]  SumOutMax=[]  SaturationOutMin=[]  SaturationOutMax=[]  PParamMin=[]  PParamMax=[]  IParamMin=[]  IParamMax=[]  DParamMin=[]  DParamMax=[]  NParamMin=[]  NParamMax=[]  KbParamMin=[]  KbParamMax=[]  KtParamMin=[]  KtParamMax=[]  KbOutMin=[]  KbOutMax=[]  KtOutMin=[]  KtOutMax=[]  IntegratorOutMin=[]  IntegratorOutMax=[]  FilterOutMin=[]  FilterOutMax=[]  SumI1OutMin=[]  SumI1OutMax=[]  SumI2OutMin=[]  SumI2OutMax=[]  SumI3OutMin=[]  SumI3OutMax=[]  SumI4OutMin=[]  SumI4OutMax=[]  SumDOutMin=[]  SumDOutMax=[]  DifferentiatorOutMin=[]  DifferentiatorOutMax=[]  FilterDiffOutCoefMin=[]  FilterDiffOutCoefMax=[]  ReciprocalOutMin=[]  ReciprocalOutMax=[]  SumDenOutMin=[]  SumDenOutMax=[]  SumNumOutMin=[]  SumNumOutMax=[]  DivideOutMin=[]  DivideOutMax=[]  UdiffTsProdOutMin=[]  UdiffTsProdOutMax=[]  NTsProdOutMin=[]  NTsProdOutMax=[]  UintegralTsProdOutMin=[]  UintegralTsProdOutMax=[]  UngainTsProdOutMin=[]  UngainTsProdOutMax=[]  ClampingZeroOutDataTypeStr=Inherit: Inherit via back propagation  ClampingZeroOutMin=[]  ClampingZeroOutMax=[]  FilterDenConstantOutDataTypeStr=Inherit: Inherit via back propagation  FilterDenConstantOutMin=[]  FilterDenConstantOutMax=[]  PCopyOutDataTypeStr=Inherit: Inherit via back propagation  PCopyOutMin=[]  PCopyOutMax=[]  NCopyOutDataTypeStr=Inherit: Inherit via back propagation  NCopyOutMin=[]  NCopyOutMax=[]  IntegratorContinuousStateAttributes=''  IntegratorStateMustResolveToSignalObject=off  IntegratorRTWStateStorageClass=Auto  FilterContinuousStateAttributes=''  FilterStateMustResolveToSignalObject=off  FilterRTWStateStorageClass=Auto  ParallelPVariant=InternalParameters  IdealPVariant=Disabled  IVariant=InternalParameters  DVariant=InternalParameters  IntegratorVariant=Continuous  SatVariant=Disabled  AWVariant=Passthrough  PCopyVariant=Disabled  TRVariant=Disabled  FdbkBlocksVariant=Forward  IdealPFdbkVariant=Disabled  SatFdbkVariant=Disabled  DerivativeFilterVariant=ContFilter  NVariant=InternalParameters  NCopyVariant=Disabled  FilterICVariant=InternalICsFilter  IntegratorICVariant=InternalICs  ExternalResetVariant=Disabled  TRSumVariant=Passthrough  SumFdbkVariant=Disabled  SumVariant=Sum_PID  TsampFilterVariant=InternalTs  TsampNgainVariant=Passthrough  TsampIntegralVariant=Disabled_SignalSpec  ExternalSaturationOutDataTypeStr=Inherit: Same as second input
  Radians to Degrees : simulink_extras/Transformations/Radians to Degrees
  Saturation : Saturate  UpperLimit=1  LowerLimit=-1
  Sum : Sum  Inputs=|+-
  Yaw Control : Outport
  wires:
  Target Yaw/1 -> Sum/1
  Sum/1 -> PID Controller/1
  PID Controller/1 -> Saturation/1
  Saturation/1 -> Yaw Control/1
  Current Yaw/1 -> Radians to Degrees/1
  Radians to Degrees/1 -> Sum/2

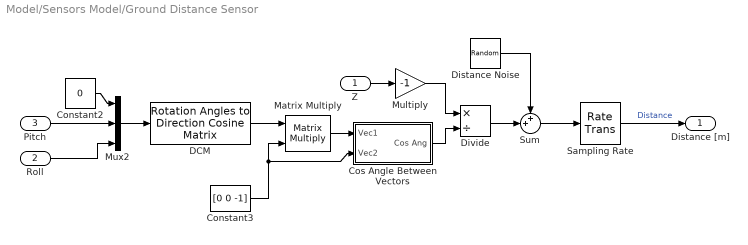
== system Model/Sensors Model/Ground Distance Sensor ==
  Z : Inport
  Roll : Inport  Port=2
  Pitch : Inport  Port=3
  Constant2 : Constant  Value=0
  Constant3 : Constant  Value=[0 0 -1]
  Cos Angle Between Vectors : Subsystem
  DCM : sharedtransform/Rotation Angles to Direction Cosine Matrix  rotationOrder=ZYX  aMode=aMode
  Distance Noise : RandomNumber  Variance=0.0005  SampleTime=0.1
  Divide : Product  Inputs=*/
  Matrix Multiply : Product  Multiplication=Matrix(*)
  Multiply : Gain  Gain=-1
  Mux2 : Mux  Inputs=3
  Sampling Rate : RateTransition  OutPortSampleTime=0.05
  Sum : Sum  Inputs=++|
  Distance [m] : Outport
  wires:
  Cos Angle Between Vectors/1(Cos Ang) -> Divide/2
  Z/1 -> Multiply/1
  Sampling Rate/1 -> Distance [m]/1  "Distance"
  Multiply/1 -> Divide/1
  Divide/1 -> Sum/2
  Sum/1 -> Sampling Rate/1
  Distance Noise/1 -> Sum/1
  DCM/1 -> Matrix Multiply/1
  Constant2/1 -> Mux2/1
  Mux2/1 -> DCM/1
  Pitch/1 -> Mux2/2
  Roll/1 -> Mux2/3
  Constant3/1 -> Matrix Multiply/2, Cos Angle Between Vectors/2(Vec2)
  Matrix Multiply/1 -> Cos Angle Between Vectors/1(Vec1)

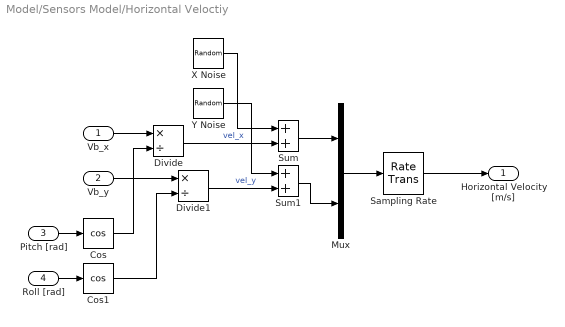
== system Model/Sensors Model/Horizontal Veloctiy ==
  Vb_x : Inport
  Vb_y : Inport  Port=2
  Pitch [rad] : Inport  Port=3
  Roll [rad] : Inport  Port=4
  Cos : Trigonometry  Operator=cos
  Cos1 : Trigonometry  Operator=cos
  Divide : Product  Inputs=*/
  Divide1 : Product  Inputs=*/
  Mux : Mux  Inputs=2
  Sampling Rate : RateTransition  OutPortSampleTime=0.1
  Sum : Sum
  Sum1 : Sum
  X Noise : RandomNumber  Variance=.01  Seed=546456  SampleTime=0.1
  Y Noise : RandomNumber  Variance=.01  Seed=4325342  SampleTime=0.1
  Horizontal Velocity [m/s] : Outport
  wires:
  Sum1/1 -> Mux/2
  X Noise/1 -> Sum/1
  Sum/1 -> Mux/1
  Y Noise/1 -> Sum1/1
  Mux/1 -> Sampling Rate/1
  Sampling Rate/1 -> Horizontal Velocity [m/s]/1
  Vb_x/1 -> Divide/1
  Divide/1 -> Sum/2  "vel_x"
  Vb_y/1 -> Divide1/1
  Divide1/1 -> Sum1/2  "vel_y"
  Pitch [rad]/1 -> Cos/1
  Roll [rad]/1 -> Cos1/1
  Cos/1 -> Divide/2
  Cos1/1 -> Divide1/2

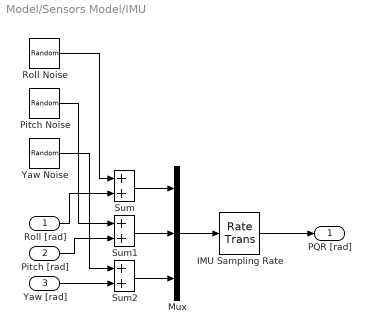
== system Model/Sensors Model/IMU ==
  Roll [rad] : Inport
  Pitch [rad] : Inport  Port=2
  Yaw [rad] : Inport  Port=3
  IMU Sampling Rate : RateTransition  OutPortSampleTime=0.01
  Mux : Mux  Inputs=3
  Pitch Noise : RandomNumber  Variance=.00005  Seed=4325342  SampleTime=0.1
  Roll Noise : RandomNumber  Variance=.00005  Seed=546456  SampleTime=0.1
  Sum : Sum
  Sum1 : Sum
  Sum2 : Sum
  Yaw Noise : RandomNumber  Variance=.00005  Seed=32454634  SampleTime=0.1
  PQR [rad] : Outport
  wires:
  Yaw Noise/1 -> Sum2/1
  Sum1/1 -> Mux/2
  Roll Noise/1 -> Sum/1
  Sum2/1 -> Mux/3
  Sum/1 -> Mux/1
  Pitch Noise/1 -> Sum1/1
  Mux/1 -> IMU Sampling Rate/1
  IMU Sampling Rate/1 -> PQR [rad]/1
  Yaw [rad]/1 -> Sum2/2
  Pitch [rad]/1 -> Sum1/2
  Roll [rad]/1 -> Sum/2

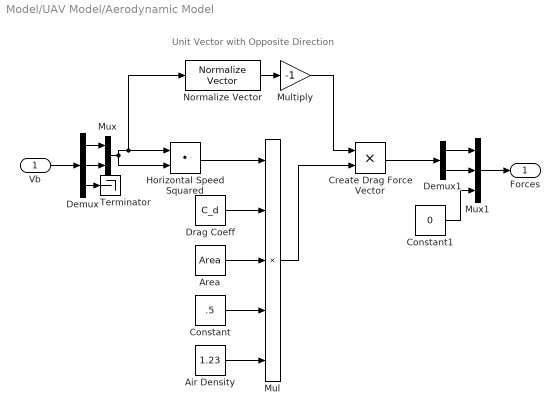
== system Model/UAV Model/Aerodynamic Model ==
  note: Unit Vector with Opposite Direction
  Vb : Inport
  Air Density : Constant  Value=1.23
  Area : Constant  Value=Area
  Constant : Constant  Value=.5
  Constant1 : Constant  Value=0
  Create Drag Force Vector : Product  Inputs=**
  Demux : Demux  Outputs=3
  Demux1 : Demux  Outputs=2
  Drag Coeff : Constant  Value=C_d
  Horizontal Speed Squared : DotProduct  OutDataTypeStr=Inherit: Inherit via internal rule
  Mul : Product  Inputs=*****
  Multiply : Gain  Gain=-1
  Mux : Mux  Inputs=2
  Mux1 : Mux  Inputs=3
  Normalize Vector : vrlib/Utilities/Normalize Vector  maxzero=0
  Terminator : Terminator
  Forces : Outport
  wires:
  Vb/1 -> Demux/1
  Demux/3 -> Terminator/1
  Demux/1 -> Mux/1
  Demux/2 -> Mux/2
  Normalize Vector/1 -> Multiply/1
  Mux/1 -> Horizontal Speed Squared/2, Normalize Vector/1, Horizontal Speed Squared/1
  Horizontal Speed Squared/1 -> Mul/1
  Drag Coeff/1 -> Mul/2
  Area/1 -> Mul/3
  Constant/1 -> Mul/4
  Air Density/1 -> Mul/5
  Multiply/1 -> Create Drag Force Vector/1
  Mul/1 -> Create Drag Force Vector/2
  Mux1/1 -> Forces/1
  Demux1/1 -> Mux1/1
  Demux1/2 -> Mux1/2
  Create Drag Force Vector/1 -> Demux1/1
  Constant1/1 -> Mux1/3

== system Model/UAV Model/Gravity ==
  DCM_be : Inport
  Mass : Inport  Port=2
  Divide : Product  Inputs=**
  Gravity : Constant  Value=[0 0 9.81]
  Matrix Multiply : Product  Multiplication=Matrix(*)
  Gravity_Body [N] : Outport
  wires:
  Matrix Multiply/1 -> Gravity_Body [N]/1
  DCM_be/1 -> Matrix Multiply/1
  Gravity/1 -> Divide/1
  Divide/1 -> Matrix Multiply/2
  Mass/1 -> Divide/2

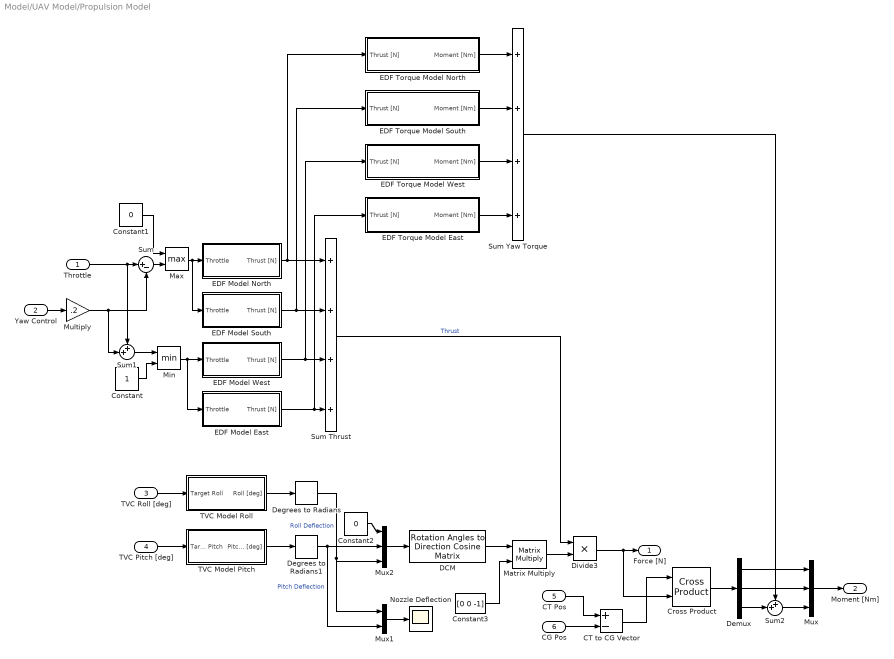
== system Model/UAV Model/Propulsion Model ==
  Throttle : Inport
  Yaw Control : Inport  Port=2
  TVC Roll [deg] : Inport  Port=3
  TVC Pitch [deg] : Inport  Port=4
  CT Pos : Inport  Port=5
  CG Pos : Inport  Port=6
  CT to CG Vector : Sum  Inputs=+-
  Constant : Constant
  Constant1 : Constant  Value=0
  Constant2 : Constant  Value=0
  Constant3 : Constant  Value=[0 0 -1]
  Cross Product : matrix_library/Cross Product
  DCM : sharedtransform/Rotation Angles to Direction Cosine Matrix  rotationOrder=ZYX  aMode=aMode
  Degrees to Radians : simulink_extras/Transformations/Degrees to Radians
  Degrees to Radians1 : simulink_extras/Transformations/Degrees to Radians
  Demux : Demux  Outputs=3
  Divide3 : Product  Inputs=**
  EDF Model East : Subsystem
  EDF Model North : Subsystem
  EDF Model South : Subsystem
  EDF Model West : Subsystem
  EDF Torque Model East : Subsystem
  EDF Torque Model North : Subsystem
  EDF Torque Model South : Subsystem
  EDF Torque Model West : Subsystem
  Matrix Multiply : Product  Multiplication=Matrix(*)
  Max : MinMax  Function=max  Inputs=2
  Min : MinMax  Inputs=2
  Multiply : Gain  Gain=.2
  Mux : Mux  Inputs=3
  Mux1 : Mux  Inputs=2
  Mux2 : Mux  Inputs=3
  Nozzle Deflection : Scope
  Sum : Sum  Inputs=|+-
  Sum Thrust : Sum  Inputs=++++
  Sum Yaw Torque : Sum  Inputs=++++
  Sum1 : Sum  Inputs=++|
  Sum2 : Sum  Inputs=++|
  TVC Model Pitch : Subsystem
  TVC Model Roll : Subsystem
  Force [N] : Outport
  Moment [Nm] : Outport  Port=2
  wires:
  TVC Roll [deg]/1 -> TVC Model Roll/1(Target Roll)
  EDF Model West/1(Thrust [N]) -> EDF Torque Model West/1(Thrust [N]), Sum Thrust/3
  EDF Model South/1(Thrust [N]) -> EDF Torque Model South/1(Thrust [N]), Sum Thrust/2
  EDF Model North/1(Thrust [N]) -> EDF Torque Model North/1(Thrust [N]), Sum Thrust/1
  EDF Model East/1(Thrust [N]) -> EDF Torque Model East/1(Thrust [N]), Sum Thrust/4
  TVC Pitch [deg]/1 -> TVC Model Pitch/1(Target Pitch)
  TVC Model Roll/1(Roll [deg]) -> Degrees to Radians/1
  TVC Model Pitch/1(Pitch [deg]) -> Degrees to Radians1/1
  Degrees to Radians/1 -> Mux1/1, Mux2/3  "Roll Deflection"
  Degrees to Radians1/1 -> Mux1/2, Mux2/2  "Pitch Deflection"
  Divide3/1 -> Cross Product/2, Force [N]/1
  Sum Thrust/1 -> Divide3/1  "Thrust"
  Mux/1 -> Moment [Nm]/1
  EDF Torque Model North/1(Moment [Nm]) -> Sum Yaw Torque/1
  EDF Torque Model South/1(Moment [Nm]) -> Sum Yaw Torque/2
  EDF Torque Model West/1(Moment [Nm]) -> Sum Yaw Torque/3
  EDF Torque Model East/1(Moment [Nm]) -> Sum Yaw Torque/4
  Yaw Control/1 -> Multiply/1
  Multiply/1 -> Sum1/2, Sum/2
  Throttle/1 -> Sum/1, Sum1/1
  Min/1 -> EDF Model East/1(Throttle), EDF Model West/1(Throttle)
  Sum1/1 -> Min/1
  Constant/1 -> Min/2
  Max/1 -> EDF Model South/1(Throttle), EDF Model North/1(Throttle)
  Sum/1 -> Max/2
  Constant1/1 -> Max/1
  Mux1/1 -> Nozzle Deflection/1
  Mux2/1 -> DCM/1
  Constant2/1 -> Mux2/1
  DCM/1 -> Matrix Multiply/1
  Constant3/1 -> Matrix Multiply/2
  Matrix Multiply/1 -> Divide3/2
  CG Pos/1 -> CT to CG Vector/2
  CT Pos/1 -> CT to CG Vector/1
  CT to CG Vector/1 -> Cross Product/1
  Cross Product/1 -> Demux/1
  Demux/1 -> Mux/1
  Demux/2 -> Mux/2
  Demux/3 -> Sum2/2
  Sum2/1 -> Mux/3
  Sum Yaw Torque/1 -> Sum2/1

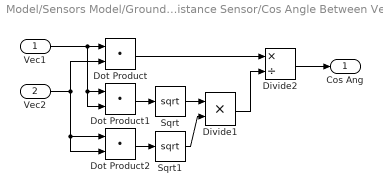
== system Model/Sensors Model/Ground Distance Sensor/Cos Angle Between Vectors ==
  Vec1 : Inport
  Vec2 : Inport  Port=2
  Divide1 : Product  Inputs=**
  Divide2 : Product  Inputs=*/
  Dot Product : DotProduct  OutDataTypeStr=Inherit: Inherit via internal rule
  Dot Product1 : DotProduct  OutDataTypeStr=Inherit: Inherit via internal rule
  Dot Product2 : DotProduct  OutDataTypeStr=Inherit: Inherit via internal rule
  Sqrt : Sqrt
  Sqrt1 : Sqrt
  Cos Ang : Outport
  wires:
  Vec1/1 -> Dot Product1/2, Dot Product1/1, Dot Product/1
  Dot Product/1 -> Divide2/1
  Dot Product2/1 -> Sqrt1/1
  Vec2/1 -> Dot Product2/2, Dot Product2/1, Dot Product/2
  Divide1/1 -> Divide2/2
  Dot Product1/1 -> Sqrt/1
  Sqrt1/1 -> Divide1/2
  Sqrt/1 -> Divide1/1
  Divide2/1 -> Cos Ang/1

== system Model/UAV Model/Propulsion Model/EDF Model East ==
  Throttle : Inport
  EDF Transfer Fcn : TransferFcn  Numerator=[10]  Denominator=[0.25 1]
  Thrust [N] : Outport
  wires:
  Throttle/1 -> EDF Transfer Fcn/1
  EDF Transfer Fcn/1 -> Thrust [N]/1

== system Model/UAV Model/Propulsion Model/EDF Model North ==
  Throttle : Inport
  EDF Transfer Fcn : TransferFcn  Numerator=[10]  Denominator=[0.25 1]
  Thrust [N] : Outport
  wires:
  Throttle/1 -> EDF Transfer Fcn/1
  EDF Transfer Fcn/1 -> Thrust [N]/1

== system Model/UAV Model/Propulsion Model/EDF Model South ==
  Throttle : Inport
  EDF Transfer Fcn : TransferFcn  Numerator=[10]  Denominator=[0.25 1]
  Thrust [N] : Outport
  wires:
  Throttle/1 -> EDF Transfer Fcn/1
  EDF Transfer Fcn/1 -> Thrust [N]/1

== system Model/UAV Model/Propulsion Model/EDF Model West ==
  Throttle : Inport
  EDF Transfer Fcn : TransferFcn  Numerator=[10]  Denominator=[0.25 1]
  Thrust [N] : Outport
  wires:
  Throttle/1 -> EDF Transfer Fcn/1
  EDF Transfer Fcn/1 -> Thrust [N]/1

== system Model/UAV Model/Propulsion Model/EDF Torque Model East ==
  note: Make acutal thrust/torque relation here
  Thrust [N] : Inport
  Multiply : Gain  Gain=0.01
  Moment [Nm] : Outport
  wires:
  Thrust [N]/1 -> Multiply/1
  Multiply/1 -> Moment [Nm]/1

== system Model/UAV Model/Propulsion Model/EDF Torque Model North ==
  note: Make acutal thrust/torque relation here
  Thrust [N] : Inport
  Multiply : Gain  Gain=-0.01
  Moment [Nm] : Outport
  wires:
  Thrust [N]/1 -> Multiply/1
  Multiply/1 -> Moment [Nm]/1

== system Model/UAV Model/Propulsion Model/EDF Torque Model South ==
  note: Make acutal thrust/torque relation here
  Thrust [N] : Inport
  Multiply : Gain  Gain=-0.01
  Moment [Nm] : Outport
  wires:
  Thrust [N]/1 -> Multiply/1
  Multiply/1 -> Moment [Nm]/1

== system Model/UAV Model/Propulsion Model/EDF Torque Model West ==
  note: Make acutal thrust/torque relation here
  Thrust [N] : Inport
  Multiply : Gain  Gain=0.01
  Moment [Nm] : Outport
  wires:
  Thrust [N]/1 -> Multiply/1
  Multiply/1 -> Moment [Nm]/1

== system Model/UAV Model/Propulsion Model/TVC Model Pitch ==
  Target Pitch : Inport
  Gimball Pitch Transfer Fcn : TransferFcn  Denominator=[0.25 1]
  Pitch [deg] : Outport
  wires:
  Target Pitch/1 -> Gimball Pitch Transfer Fcn/1
  Gimball Pitch Transfer Fcn/1 -> Pitch [deg]/1

== system Model/UAV Model/Propulsion Model/TVC Model Roll ==
  Target Roll : Inport
  Gimball Roll Transfer Fcn : TransferFcn  Denominator=[0.25 1]
  Roll [deg] : Outport
  wires:
  Target Roll/1 -> Gimball Roll Transfer Fcn/1
  Gimball Roll Transfer Fcn/1 -> Roll [deg]/1
